simulink model "Reset_timer"  (Simulink 5.0)
settings: Solver=ode45  StartTime=0.0  StopTime=.1  MaxStep=.00001  RelTol=1e-6
settings Model: LastModifiedBy=ravi

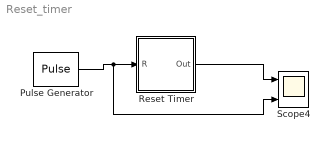
== system Reset_timer ==
  Pulse Generator : DiscretePulseGenerator  PulseType=Time based  Period=.00011  PulseWidth=50
  Reset Timer : Subsystem
  Scope4 : Scope  NumInputPorts=2
      settings: TimeRange=0.0333  YMin=-5~-5  YMax=5~5  MaxDataPoints=500000
  wires:
  Pulse Generator/1 -> Reset Timer/1(R), Scope4/2
  Reset Timer/1(Out) -> Scope4/1

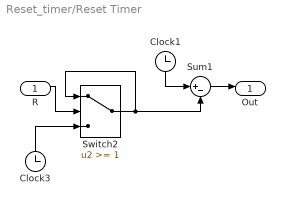
== system Reset_timer/Reset Timer ==
  R : Inport
  Clock1 : Clock
      settings: Orientation=down  Decimation=10
  Clock3 : Clock
      settings: Orientation=up  Decimation=4
  Sum1 : Sum  Inputs=|+-  SaturateOnIntegerOverflow=on  InputSameDT=on
  Switch2 : Switch  Threshold=1  ShowAdditionalParam=on  RndMeth=Zero
  Out : Outport
  wires:
  Clock1/1 -> Sum1/1
  Clock3/1 -> Switch2/3
  Switch2/1 -> Switch2/1, Sum1/2
  Sum1/1 -> Out/1
  R/1 -> Switch2/2
